simulink model "model_bez"  (R2015a)
settings: Solver=ode3  StartTime=0.0  StopTime=10.0  FixedStep=0.001  RelTol=1e-3
values from neighbouring files (symbols this model uses):
  K = 1    [Helicopter_main.m]    (also in cel_bez.m = params(2); identyfikacja_moment_bez.m)
  offset = 28.13    [cel_bez.m]    (also in identyfikacja_moment_bez.m = 27.13)
  psi = 0.0125    [Helicopter_main.m]    (also in cel_bez.m = params(1); identyfikacja_moment_bez.m)
  T = 0.4495    [Helicopter_main.m]    (also in cel_bez.m = params(3); char_U_V_Az.m = 6; char_U_V_Pitch.m = 6; identyfikacja_moment_bez.m)
settings Model: Creator=Student  LastModifiedBy=Student

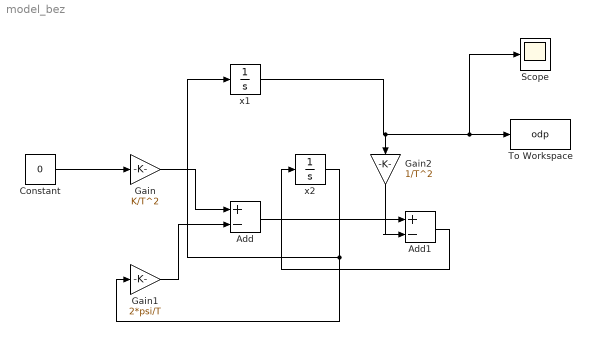
== system model_bez ==
  Add : Sum  Inputs=+-
  Add1 : Sum  Inputs=+-
  Constant : Constant  Value=0
  Gain : Gain  Gain=K/T^2
  Gain1 : Gain  Gain=2*psi/T
  Gain2 : Gain  Gain=1/T^2
  Scope : Scope
  To Workspace : ToWorkspace  VariableName=odp  SampleTime=-1
  x1 : Integrator  InitialCondition=offset
  x2 : Integrator
  wires:
  Gain/1 -> Add/1
  Constant/1 -> Gain/1
  Gain1/1 -> Add/2
  x2/1 -> x1/1, Gain1/1
  Add/1 -> Add1/1
  Add1/1 -> x2/1
  x1/1 -> Scope/1, To Workspace/1, Gain2/1
  Gain2/1 -> Add1/2
